simulink model "project_2_ass"  (R2019a)
settings: Solver=VariableStepAuto  StartTime=0.0  StopTime=10.0  RelTol=1e-3
libraries: simulink x1
settings Model: Creator=Nikita  LastModifiedBy=Nikita

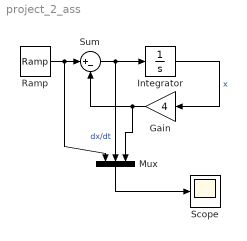
== system project_2_ass ==
  Gain : Gain  Gain=4
  Integrator : Integrator
  Mux : Mux  Inputs=3
  Ramp : simulink/Sources/Ramp  slope=u  start=0  InitialOutput=0
  Scope : Scope
  Sum : Sum  Inputs=|+-
  wires:
  Gain/1 -> Mux/3, Sum/2
  Sum/1 -> Mux/2, Integrator/1  "dx/dt"
  Integrator/1 -> Gain/1  "x"
  Ramp/1 -> Mux/1, Sum/1
  Mux/1 -> Scope/1
